simulink model "MotorXplorer1"  (R2024b)
settings: Solver=FixedStepAuto  StartTime=0.0  StopTime=inf  FixedStep=0.01  RelTol=1e-3
undefined symbols (not defined in the file): Blocking, LF, Non
libraries: hdlsllib x5, amg_usbconverter_n_connect_lib x3
settings Model: Creator=beamk  LastModifiedBy=bpbeam

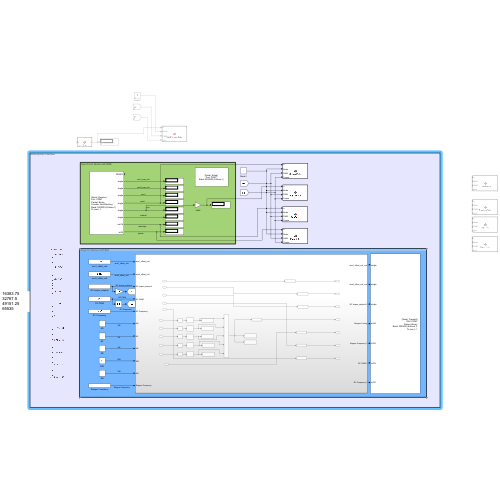
[thumbnail: Simulink's stored preview of the top-level diagram]
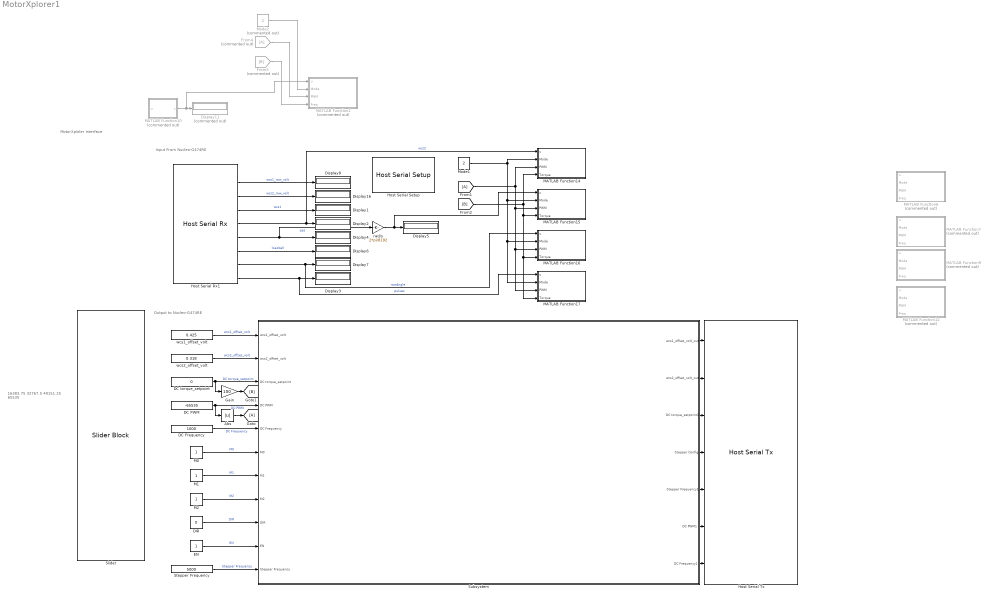
== system MotorXplorer1 ==
  note: 16383.75
      | 32767.5
      | 49151.25
      | 65535
  note: Output to Nucleo-G474RE
  note: Input From Nucleo-G474RE
  note: MotorXploler Interface
  Abs : Abs  SaturateOnIntegerOverflow=off
  DC Frequency : Constant  Value=1000
  DC PWM : Constant  Value=-65535
  DC torque_setpoint : Constant  Value=0
  DIR : Constant  Value=0  OutDataTypeStr=uint8
  Display{1..8,16} (9 alike) : Display
  Display11 : Display  Commented=on
  EN : Constant  OutDataTypeStr=uint8
  From1 : From
  From4 : From  Commented=on
  From5 : From  Commented=on  GotoTag=B
  Gain : Gain  Gain=100
  Goto : Goto
  Host Serial Rx1 : amg_usbconverter_n_connect_lib/Host Serial Rx  conf=rx  port=<auto>  baudrate=2000000  databits=8  parity=None  stopbit=1  flowcontrol=None  transfer=Non-Blocking  timeout=5  packetmode=Binary  enableinitialvalues=off  initialvalues=[]  binheader='45'  binterminator='A'  porttype_double=0  porttype_single=6  porttype_int8=0  porttype_uint8=0  porttype_int16=0  porttype_uint16=1  porttype_int32=1  porttype_uint32=0  asciiformat='%f,%f,%d,%d'  rx_asciiterminator="LF (0x0A - \"\\n\")"  tx_asciiterminator="CRLF (0x0D 0x0A - \"\\r\\n\")"  sampletime=-1  enablecustomportlabel=off  cinputportlabel=0  coutputportlabel=A  portpinstr=0  blockid=HostSerialRx1  inputporttype=[]  inputportwidth=[]  inputportlabel={}  outputporttype=[3 1 1 1 1 1 1 5 6]  outputportwidth=[1 1 1 1 1 1 1 1 1]  outputportlabel={'READY','single','single','single','single','single','single','uint16','int32'}  compat=0  optionstring=[]  autoport='COM7'
  Host Serial Setup : amg_usbconverter_n_connect_lib/Host Serial Setup  conf=setup  port=<auto>  baudrate=2000000  databits=8  parity=None  stopbit=1  flowcontrol=None  transfer=Blocking  timeout=2  packetmode=Binary  initialvalues=[]  binheader='7E 7E'  binterminator='03 03'  porttype_double=0  porttype_single=1  porttype_int8=0  porttype_uint8=0  porttype_int16=0  porttype_uint16=0  porttype_int32=0  porttype_uint32=2  asciiformat='%d %u %x'  rx_asciiterminator="CRLF (0x0D 0x0A - \"\\r\\n\")"  tx_asciiterminator="CRLF (0x0D 0x0A - \"\\r\\n\")"  sampletime=-1  enablecustomportlabel=off  cinputportlabel=0  coutputportlabel=A  portpinstr=0  blockid=HostSerialSetup  inputporttype=[]  inputportwidth=[]  inputportlabel={}  outputporttype=[]  outputportwidth=[]  outputportlabel={}  compat=0  optionstring=[]  autoport='COM7'
  Host Serial Tx : amg_usbconverter_n_connect_lib/Host Serial Tx  conf=tx  port=<auto>  baudrate=2000000  databits=8  parity=None  stopbit=1  flowcontrol=None  transfer=Blocking  timeout=2  packetmode=Binary  initialvalues=[]  binheader='45'  binterminator='A'  porttype_double=0  porttype_single=3  porttype_int8=0  porttype_uint8=1  porttype_int16=0  porttype_uint16=0  porttype_int32=3  porttype_uint32=0  asciiformat='%d,%f'  rx_asciiterminator="CRLF (0x0D 0x0A - \"\\r\\n\")"  tx_asciiterminator="CRLF (0x0D 0x0A - \"\\r\\n\")"  sampletime=-1  enablecustomportlabel=off  cinputportlabel=0  coutputportlabel=A  portpinstr=0  blockid=HostSerialTx  inputporttype=[1 1 1 3 6 6 6]  inputportwidth=[1 1 1 1 1 1 1]  inputportlabel={'single','single','single','uint8','int32','int32','int32'}  outputporttype=[]  outputportwidth=[]  outputportlabel={}  compat=0  optionstring=[]  autoport='COM7'
      settings: SourceProductName=aMG USB Converter N
  M0 : Constant  OutDataTypeStr=uint8
  M1 : Constant  OutDataTypeStr=uint8
  M2 : Constant  OutDataTypeStr=uint8
  MATLAB Function10 : MATLAB Function  Commented=on  TreatAsAtomicUnit=on
  MATLAB Function12 : MATLAB Function  Commented=on  TreatAsAtomicUnit=on
  MATLAB Function14 : MATLAB Function  TreatAsAtomicUnit=on
  MATLAB Function15 : MATLAB Function  TreatAsAtomicUnit=on
  MATLAB Function16 : MATLAB Function  TreatAsAtomicUnit=on
  MATLAB Function17 : MATLAB Function  TreatAsAtomicUnit=on
  MATLAB Function2 : MATLAB Function  Commented=on  TreatAsAtomicUnit=on
  MATLAB Function6 : MATLAB Function  Commented=on  TreatAsAtomicUnit=on
  MATLAB Function7 : MATLAB Function  Commented=on  TreatAsAtomicUnit=on
  MATLAB Function9 : MATLAB Function  Commented=on  TreatAsAtomicUnit=on
  Mode1 : Constant  Value=2  OutDataTypeStr=int32
  Mode2 : Constant  Commented=on  Value=2  OutDataTypeStr=int32
  Slider : SliderBlock  ScaleMin=-65535  ScaleMax=65535
  Stepper Frequency : Constant  Value=5000
  Subsystem : Subsystem
  rad/s : Gain  Gain=2*pi/8192
  wcs1_offset_volt : Constant  Value=0.425  OutDataTypeStr=single
  wcs2_offset_volt : Constant  Value=0.318  OutDataTypeStr=single
  wires:
  Host Serial Rx1/2 -> Display8/1  "wcs1_raw_volt"
  Host Serial Rx1/3 -> Display16/1  "wcs2_raw_volt"
  Host Serial Rx1/7 -> Display6/1  "loadcell"
  Host Serial Rx1/5 -> MATLAB Function14/1(u), Display2/1  "wcs2"
  Host Serial Rx1/6 -> Display4/1, rad/s/1  "pps"
  Host Serial Rx1/4 -> Display1/1  "wcs1"
  wcs1_offset_volt/1 -> Subsystem/1(wcs1_offset_volt)  "wcs1_offset_volt"
  wcs2_offset_volt/1 -> Subsystem/2(wcs2_offset_volt)  "wcs2_offset_volt"
  DC torque_setpoint/1 -> Gain/1, Subsystem/3(DC torque_setpoint)  "DC torque_setpoint"
  DC PWM/1 -> Abs/1, Subsystem/4(DC PWM)  "DC PWM"
  DC Frequency/1 -> Subsystem/5(DC Frequency)  "DC Frequency"
  M0/1 -> Subsystem/6(M0)  "M0"
  M1/1 -> Subsystem/7(M1)  "M1"
  M2/1 -> Subsystem/8(M2)  "M2"
  DIR/1 -> Subsystem/9(DIR)  "DIR"
  EN/1 -> Subsystem/10(EN)  "EN"
  Stepper Frequency/1 -> Subsystem/11(Stepper Frequency)  "Stepper Frequency"
  Subsystem/1(wcs1_offset_volt_out) -> Host Serial Tx/1
  Subsystem/2(wcs2_offset_volt_out) -> Host Serial Tx/2
  Subsystem/3(DC torque_setpoint1) -> Host Serial Tx/3
  Subsystem/4(Stepper Config) -> Host Serial Tx/4
  Subsystem/5(Stepper Frequency1) -> Host Serial Tx/5
  Subsystem/6(DC PWM1) -> Host Serial Tx/6
  Subsystem/7(DC Frequency1) -> Host Serial Tx/7
  rad/s/1 -> MATLAB Function15/1(u), Display5/1
  Mode2/1 -> MATLAB Function2/2(Mode)
  Host Serial Rx1/9 -> MATLAB Function17/1(u), Display3/1  "pulses"
  Host Serial Rx1/8 -> MATLAB Function16/1(u), Display7/1  "rawAngle"
  From4/1 -> MATLAB Function2/3(PWM)
  From5/1 -> MATLAB Function2/4(Freq)
  Abs/1 -> Goto/1
  MATLAB Function10/1(v) -> MATLAB Function2/1(u), Display11/1
  Mode1/1 -> MATLAB Function17/2(Mode), MATLAB Function16/2(Mode), MATLAB Function15/2(Mode), MATLAB Function14/2(Mode)
  From1/1 -> MATLAB Function17/3(PWM), MATLAB Function16/3(PWM), MATLAB Function15/3(PWM), MATLAB Function14/3(PWM)
  [B] -> MATLAB Function17/4(Torque), MATLAB Function16/4(Torque), MATLAB Function15/4(Torque), MATLAB Function14/4(Torque)
  Gain/1 -> [B]

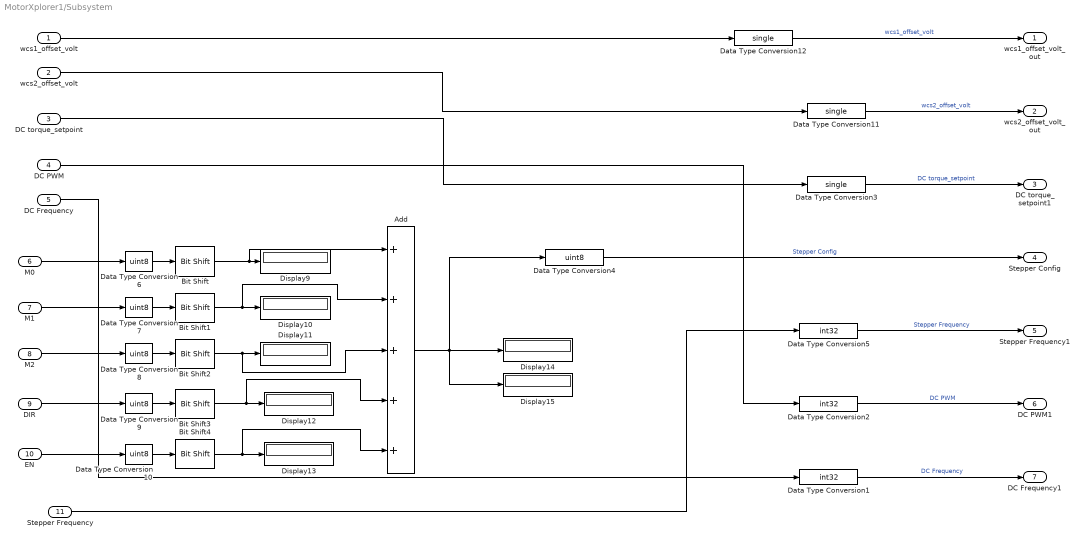
== system MotorXplorer1/Subsystem ==
  wcs1_offset_volt : Inport
  wcs2_offset_volt : Inport  Port=2
  DC torque_setpoint : Inport  Port=3
  DC PWM : Inport  Port=4
  DC Frequency : Inport  Port=5
  M0 : Inport  Port=6
  M1 : Inport  Port=7
  M2 : Inport  Port=8
  DIR : Inport  Port=9
  EN : Inport  Port=10
  Stepper Frequency : Inport  Port=11
  Add : Sum  Inputs=+++++
  Bit Shift : hdlsllib/Logic and Bit Operations/Bit Shift  mode=Shift Left Logical  N=4
  Bit Shift1 : hdlsllib/Logic and Bit Operations/Bit Shift  mode=Shift Left Logical  N=3
  Bit Shift2 : hdlsllib/Logic and Bit Operations/Bit Shift  mode=Shift Left Logical  N=2
  Bit Shift3 : hdlsllib/Logic and Bit Operations/Bit Shift  mode=Shift Left Logical  N=1
  Bit Shift4 : hdlsllib/Logic and Bit Operations/Bit Shift  mode=Shift Left Logical  N=0
  Data Type Conversion1 : DataTypeConversion  OutDataTypeStr=int32  SaturateOnIntegerOverflow=off  RndMeth=Floor
  Data Type Conversion{4,6..10} (6 alike) : DataTypeConversion  OutDataTypeStr=uint8  SaturateOnIntegerOverflow=off  RndMeth=Floor
  Data Type Conversion11 : DataTypeConversion  OutDataTypeStr=single  SaturateOnIntegerOverflow=off  RndMeth=Floor
  Data Type Conversion12 : DataTypeConversion  OutDataTypeStr=single  SaturateOnIntegerOverflow=off  RndMeth=Floor
  Data Type Conversion2 : DataTypeConversion  OutDataTypeStr=int32  SaturateOnIntegerOverflow=off  RndMeth=Floor
  Data Type Conversion3 : DataTypeConversion  OutDataTypeStr=single  SaturateOnIntegerOverflow=off  RndMeth=Floor
  Data Type Conversion5 : DataTypeConversion  OutDataTypeStr=int32  SaturateOnIntegerOverflow=off  RndMeth=Floor
  Display{9..15} (7 alike) : Display
      Display10 settings: Format=binary (Stored Integer)
      Display11 settings: Format=binary (Stored Integer)
      Display12 settings: Format=binary (Stored Integer)
      Display13 settings: Format=binary (Stored Integer)
      Display14 settings: Format=binary (Stored Integer)
      Display9 settings: Format=binary (Stored Integer)
  wcs1_offset_volt_out : Outport
  wcs2_offset_volt_out : Outport  Port=2
  DC torque_setpoint1 : Outport  Port=3
  Stepper Config : Outport  Port=4
  Stepper Frequency1 : Outport  Port=5
  DC PWM1 : Outport  Port=6
  DC Frequency1 : Outport  Port=7
  wires:
  Bit Shift/1 -> Display9/1, Add/1
  Data Type Conversion8/1 -> Bit Shift2/1
  EN/1 -> Data Type Conversion10/1
  Data Type Conversion6/1 -> Bit Shift/1
  DC torque_setpoint/1 -> Data Type Conversion3/1
  Data Type Conversion2/1 -> DC PWM1/1  "DC PWM"
  Data Type Conversion7/1 -> Bit Shift1/1
  Data Type Conversion10/1 -> Bit Shift4/1
  DC PWM/1 -> Data Type Conversion2/1
  Bit Shift3/1 -> Display12/1, Add/4
  Data Type Conversion12/1 -> wcs1_offset_volt_out/1  "wcs1_offset_volt"
  Add/1 -> Display15/1, Display14/1, Data Type Conversion4/1
  Bit Shift2/1 -> Display11/1, Add/3
  Stepper Frequency/1 -> Data Type Conversion5/1
  M1/1 -> Data Type Conversion7/1
  Bit Shift1/1 -> Display10/1, Add/2
  Bit Shift4/1 -> Display13/1, Add/5
  M0/1 -> Data Type Conversion6/1
  Data Type Conversion9/1 -> Bit Shift3/1
  Data Type Conversion11/1 -> wcs2_offset_volt_out/1  "wcs2_offset_volt"
  M2/1 -> Data Type Conversion8/1
  wcs1_offset_volt/1 -> Data Type Conversion12/1
  DC Frequency/1 -> Data Type Conversion1/1
  wcs2_offset_volt/1 -> Data Type Conversion11/1
  Data Type Conversion1/1 -> DC Frequency1/1  "DC Frequency"
  DIR/1 -> Data Type Conversion9/1
  Data Type Conversion4/1 -> Stepper Config/1  "Stepper Config"
  Data Type Conversion3/1 -> DC torque_setpoint1/1  "DC torque_setpoint"
  Data Type Conversion5/1 -> Stepper Frequency1/1  "Stepper Frequency"

== matlab function MotorXplorer1/MATLAB Function2 ==
  data: u input; Mode input; PWM input; Freq input
function StallTorqueData(u, Mode, PWM, Freq)
    % Convert Mode and Freq to strings for the variable name
    varName = sprintf('StallTorque_%d_%d_%d', Mode, PWM, Freq);

    % Persistent variable to store the data
    persistent data;
    if isempty(data)
        data = [];
    end

    % Append new data
    data = [data; u];

    % Export data to the workspace with dynamic variable name
    assignin('base', varName, data);
end

== matlab function MotorXplorer1/MATLAB Function12 ==
  data: u input; Mode input; PWM input; Freq input
function PulseData(u, Mode, PWM, Freq)
    % u is the input signal
    % Mode and Freq are constant inputs used to name the workspace variable

    % Convert Mode and Freq to strings for the variable name
    varName = sprintf('Pulse_%d_%d_%d', Mode, PWM, Freq);

    % Persistent variable to store the data
    persistent data;
    if isempty(data)
        data = [];
    end

    % Append new data
    data = [data; u];

    % Limit size of data (optional, for example, 1000 rows)
    % if size(data, 1) > 1000
    %     data(1, :) = []; % Remove oldest data if exceeding the limit
    % end

    % Export data to the workspace with dynamic variable name
    assignin('base', varName, data);
end

== matlab function MotorXplorer1/MATLAB Function6 ==
  data: u input; Mode input; PWM input; Freq input
function CurrentData(u, Mode, PWM, Freq)
    % u is the input signal
    % Mode and Freq are constant inputs used to name the workspace variable

    % Convert Mode and Freq to strings for the variable name
    varName = sprintf('Current_%d_%d_%d', Mode, PWM, Freq);

    % Persistent variable to store the data
    persistent data;
    if isempty(data)
        data = [];
    end

    % Append new data
    data = [data; u];

    % Limit size of data (optional, for example, 1000 rows)
    % if size(data, 1) > 100000
    %     data(1, :) = []; % Remove oldest data if exceeding the limit
    % end

    % Export data to the workspace with dynamic variable name
    assignin('base', varName, data);
end

== matlab function MotorXplorer1/MATLAB Function7 ==
  data: u input; Mode input; PWM input; Freq input
function AngVeloData(u, Mode, PWM, Freq)
    % u is the input signal
    % Mode and Freq are constant inputs used to name the workspace variable

    % Convert Mode and Freq to strings for the variable name
    varName = sprintf('AngVelo_%d_%d_%d', Mode, PWM, Freq);

    % Persistent variable to store the data
    persistent data;
    if isempty(data)
        data = [];
    end

    % Append new data
    data = [data; u];

    % Limit size of data (optional, for example, 1000 rows)
    % if size(data, 1) > 100000
    %     data(1, :) = []; % Remove oldest data if exceeding the limit
    % end

    % Export data to the workspace with dynamic variable name
    assignin('base', varName, data);
end

== matlab function MotorXplorer1/MATLAB Function9 ==
  data: u input; Mode input; PWM input; Freq input
function AngData(u, Mode, PWM, Freq)
    % u is the input signal
    % Mode and Freq are constant inputs used to name the workspace variable

    % Convert Mode and Freq to strings for the variable name
    varName = sprintf('Ang_%d_%d_%d', Mode, PWM, Freq);

    % Persistent variable to store the data
    persistent data;
    if isempty(data)
        data = [];
    end

    % Append new data
    data = [data; u];

    % Limit size of data (optional, for example, 1000 rows)
    % if size(data, 1) > 100000
    %     data(1, :) = []; % Remove oldest data if exceeding the limit
    % end

    % Export data to the workspace with dynamic variable name
    assignin('base', varName, data);
end

== matlab function MotorXplorer1/MATLAB Function10 ==
  data: u input; v output
function v = fcn(u)
    if (u < 90)
        v = 68.66666666666667 * (u-85.5);
    else
        v = 6.931456548347613 * (u-85.5) + 140.84598123215017;
    end
end

== matlab function MotorXplorer1/MATLAB Function14 ==
  data: u input; Mode input; PWM input; Torque input
function CurrentData(u, Mode, PWM, Torque)
    % Convert Mode and Freq to strings for the variable name
    varName = sprintf('Current_%d_%d_%d', Mode, PWM, Torque);

    % Persistent variable to store the data
    persistent data;
    if isempty(data)
        data = [];
    end

    % Append new data
    data = [data; u];

    % Export data to the workspace with dynamic variable name
    assignin('base', varName, data);
end

== matlab function MotorXplorer1/MATLAB Function15 ==
  data: u input; Mode input; PWM input; Torque input
function AngVeloData(u, Mode, PWM, Torque)
    % u is the input signal
    % Mode and Freq are constant inputs used to name the workspace variable

    % Convert Mode and Freq to strings for the variable name
    varName = sprintf('AngVelo_%d_%d_%d', Mode, PWM, Torque);

    % Persistent variable to store the data
    persistent data;
    if isempty(data)
        data = [];
    end

    % Append new data
    data = [data; u];

    % Limit size of data (optional, for example, 1000 rows)
    % if size(data, 1) > 100000
    %     data(1, :) = []; % Remove oldest data if exceeding the limit
    % end

    % Export data to the workspace with dynamic variable name
    assignin('base', varName, data);
end

== matlab function MotorXplorer1/MATLAB Function16 ==
  data: u input; Mode input; PWM input; Torque input
function AngData(u, Mode, PWM, Torque)
    % u is the input signal
    % Mode and Freq are constant inputs used to name the workspace variable

    % Convert Mode and Freq to strings for the variable name
    varName = sprintf('Ang_%d_%d_%d', Mode, PWM, Torque);

    % Persistent variable to store the data
    persistent data;
    if isempty(data)
        data = [];
    end

    % Append new data
    data = [data; u];

    % Limit size of data (optional, for example, 1000 rows)
    % if size(data, 1) > 100000
    %     data(1, :) = []; % Remove oldest data if exceeding the limit
    % end

    % Export data to the workspace with dynamic variable name
    assignin('base', varName, data);
end

== matlab function MotorXplorer1/MATLAB Function17 ==
  data: u input; Mode input; PWM input; Torque input
function PulseData(u, Mode, PWM, Torque)
    % u is the input signal
    % Mode and Freq are constant inputs used to name the workspace variable

    % Convert Mode and Freq to strings for the variable name
    varName = sprintf('Pulse_%d_%d_%d', Mode, PWM, Torque);

    % Persistent variable to store the data
    persistent data;
    if isempty(data)
        data = [];
    end

    % Append new data
    data = [data; u];

    % Limit size of data (optional, for example, 1000 rows)
    % if size(data, 1) > 1000
    %     data(1, :) = []; % Remove oldest data if exceeding the limit
    % end

    % Export data to the workspace with dynamic variable name
    assignin('base', varName, data);
end
